simulink model "Dll_Caller"  (R2019b)
settings: Solver=VariableStepAuto  StartTime=0.0  StopTime=10.0  RelTol=1e-3
settings Model: Creator=sasat  LastModifiedBy=sasat

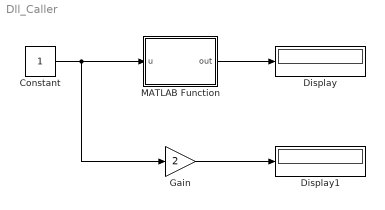
== system Dll_Caller ==
  Constant : Constant
  Display : Display
  Display1 : Display
  Gain : Gain  Gain=2
  MATLAB Function : MATLAB Function  TreatAsAtomicUnit=on
  wires:
  Constant/1 -> Gain/1, MATLAB Function/1(u)
  MATLAB Function/1(out) -> Display/1
  Gain/1 -> Display1/1

== matlab function Dll_Caller/MATLAB Function ==
  data: u input; out output
function out = fcn(u)

out = int32(0);
coder.extrinsic('loadlibrary', 'libisloaded','libpointer','calllib','unloadlibrary');

if ~libisloaded('wrapper_matlab')
    loadlibrary('wrapper_matlab.dll');
end

% libfunctionsview('wrapper_matlab')
x_ptr = libpointer('int32Ptr',u);
y_ptr = libpointer('int32Ptr',0);

[res,x,y] = calllib('wrapper_matlab','wrapper_matlab',x_ptr,y_ptr)

out = y;
unloadlibrary wrapper_matlab
